simulink model "lettura_finecorsa"  (R2017a)
settings: Solver=FixedStepAuto  StartTime=0.0  StopTime=inf  FixedStep=1e-3  RelTol=1e-3  EnableMultiTasking=on
libraries: xpcnilib x8, simulink x4
settings Model: SimulationMode=external  Creator=Davide  LastModifiedBy=Davide
settings SolverCC: EnableConcurrentExecution=on  ConcurrentTasks=on  AutoInsertRateTranBlk=on
settings DataIOCC: SaveFormat=StructureWithTime
settings OptimizationCC: BlockReduction=off  OptimizeBlockIOStorage=off  BufferReuse=off  GlobalBufferReuse=off  ExpressionFolding=off  LocalBlockOutputs=off
settings HardwareCC: ProdBitPerPointer=32  ProdBitPerSizeT=32  ProdBitPerPtrDiffT=32  ProdLargestAtomicFloat=None  ProdWordSize=32  ProdLongLongMode=on  ProdHWDeviceType=Generic->32-bit x86 compatible
settings RTWCC: SystemTargetFile=slrt.tlc  TemplateMakefile=slrt_default_tmf  Description=Simulink Real-Time  RTWCompilerOptimization=on
settings SimulinkRealTimeCC: xPCConcurrentTasks=on

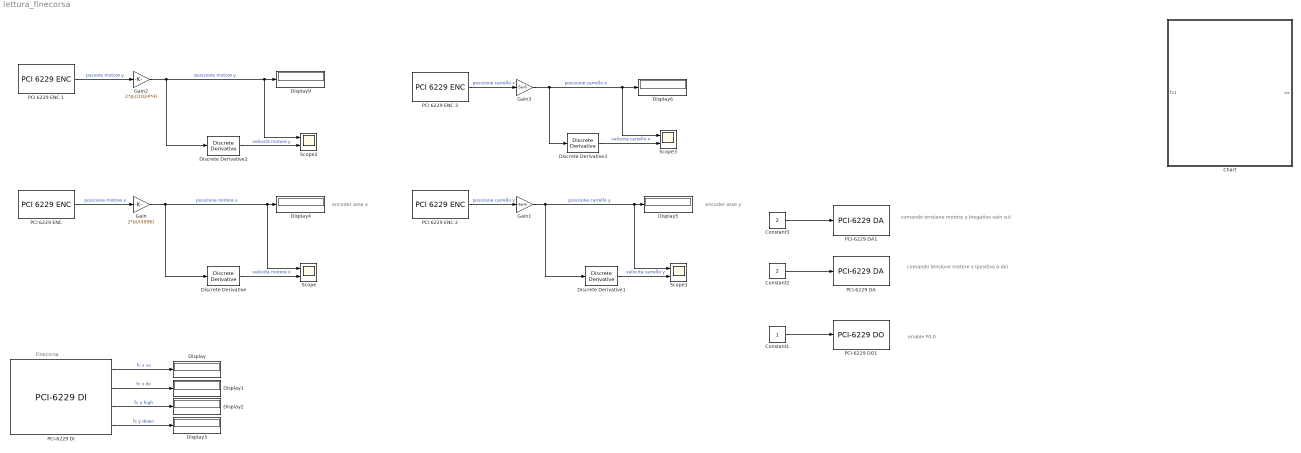
== system lettura_finecorsa ==
  note: enable P0.0
  note: comando tensione motore x (positivo a dx)
  note: comando tensione motore y (negativo vain su)
  note: Finecorsa
  note: encoder asse y
  note: encoder asse x
  Chart : Stateflow chart  TreatAsAtomicUnit=on
  Constant1 : Constant
  Constant2 : Constant  Value=2
  Constant3 : Constant  Value=2
  Discrete Derivative{,1..3} (4 alike) : simulink/Discrete/Discrete Derivative  gainval=1.0  ICPrevScaledInput=0.0  OutMin=[]  OutMax=[]  OutDataType=fixdt(1, 16)  OutScaling=2^-10  DoSatur=off
  Display{,1..6,9} (8 alike) : Display
  Gain : Gain  Gain=2*pi/(4096)
  Gain1 : Gain  Gain=-5e-6
  Gain2 : Gain  Gain=2*pi/(1024*4)
  Gain3 : Gain  Gain=-5e-6
  "PCI 6229 ENC " : xpcnilib/Incremental Encoder/PCI 6229 ENC   channel=0  countMode=Quadrature Mode x4  initCount=0  reload=on  indexPhase=A low B low  filter=None  sampleTime=0.001  slot=[4 12]
      settings: SourceProductName=Simulink Real-Time  SourceProductBaseCode=XP
  PCI 6229 ENC 1 : xpcnilib/Incremental Encoder/PCI 6229 ENC   channel=1  countMode=Quadrature Mode x4  initCount=0  reload=on  indexPhase=A low B low  filter=None  sampleTime=0.001  slot=[4 12]
      settings: SourceProductName=Simulink Real-Time  SourceProductBaseCode=XP
  PCI 6229 ENC 2 : xpcnilib/Incremental Encoder/PCI 6229 ENC   channel=0  countMode=Quadrature Mode x4  initCount=0  reload=on  indexPhase=A low B low  filter=None  sampleTime=0.001  slot=[4 15]
      settings: SourceProductName=Simulink Real-Time  SourceProductBaseCode=XP
  PCI 6229 ENC 3 : xpcnilib/Incremental Encoder/PCI 6229 ENC   channel=1  countMode=Quadrature Mode x4  initCount=0  reload=on  indexPhase=A low B low  filter=None  sampleTime=0.001  slot=[4 15]
      settings: SourceProductName=Simulink Real-Time  SourceProductBaseCode=XP
  PCI-6229 DA : xpcnilib/D//A/M Series/PCI-6229 DA  channel=[1]  reset=[1]  initValue=[0]  sampletime=0.001  slot=[4 12]
      settings: SourceProductName=Simulink Real-Time  SourceProductBaseCode=XP
  PCI-6229 DA1 : xpcnilib/D//A/M Series/PCI-6229 DA  channel=[1]  reset=[1]  initValue=[0]  sampletime=0.001  slot=[4 15]
      settings: SourceProductName=Simulink Real-Time  SourceProductBaseCode=XP
  PCI-6229 DI : xpcnilib/Digital Input/M Series/PCI-6229 DI  channel=[4 5 6 7]  sampletime=0.001  slot=[4 12]
      settings: SourceProductName=Simulink Real-Time  SourceProductBaseCode=XP
  PCI-6229 DO1 : xpcnilib/Digital Output/M Series/PCI-6229 DO  channel=[1]  reset=[1]  initValue=[0]  sampletime=0.001  slot=[4 12]
      settings: SourceProductName=Simulink Real-Time  SourceProductBaseCode=XP
  Scope{,1..3} (4 alike) : Scope  NumInputPorts=2
  wires:
  PCI-6229 DI/1 -> Display/1  "fc x sx"
  PCI-6229 DI/2 -> Display1/1  "fc x dx"
  PCI-6229 DI/3 -> Display2/1  "fc y high"
  PCI-6229 DI/4 -> Display3/1  "fc y down"
  PCI 6229 ENC 1/1 -> Gain2/1  "pozione motore y"
  PCI 6229 ENC 3/1 -> Gain3/1  "posizione carrello x"
  PCI 6229 ENC 2/1 -> Gain1/1  "posizione carrello y"
  "PCI 6229 ENC "/1 -> Gain/1  "posizione motore x"
  Discrete Derivative/1 -> Scope/2  "velocità motore x"
  Discrete Derivative1/1 -> Scope1/2  "velocità carrello y"
  Gain/1 -> Display4/1, Scope/1, Discrete Derivative/1  "posizione motore x"
  Gain1/1 -> Scope1/1, Display5/1, Discrete Derivative1/1  "posizione carrello y"
  Gain2/1 -> Scope2/1, Display9/1, Discrete Derivative2/1  "posizione motore y"
  Gain3/1 -> Discrete Derivative3/1, Scope3/1, Display6/1  "posizione carrello x"
  Constant1/1 -> PCI-6229 DO1/1
  Constant2/1 -> PCI-6229 DA/1
  Constant3/1 -> PCI-6229 DA1/1
  Discrete Derivative2/1 -> Scope2/2  "velocità motore y"
  Discrete Derivative3/1 -> Scope3/2  "velocità carrello x"

== stateflow chart lettura_finecorsa/Chart ==
  state encoder_2
    du:
    x=1;
    vx=6;
  state ?
  state encoder_1
    du:
    y=3;
  (default) -> encoder_2
  ? -> (junction 20)
  encoder_2 -> encoder_1 : [fc1==1]
  data: fc1 input; vx output
